simulink library "vmc"  (R2021b)
settings: Solver=VariableStepAuto  StartTime=0.0  StopTime=10.0  RelTol=1e-3
undefined symbols (not defined in the file or in its folder): AVMC_ACCDeltaTqIGain_X_kph, AVMC_ACCDeltaTqIGain_Y_mps2, AVMC_ACCDeltaTqPGain_X_kph, AVMC_ACCDeltaTqPGain_Y_kph, AVMC_ACCLongSteadyCtrl_X_kph, AVMC_AggressJerkPCT4AT_X_kph, AVMC_AggressJerkPCT_X_kph, AVMC_AggressLimitPCT4AT_X_kph, AVMC_AggressLimitPCT_X_kph, AVMC_CCLongSteadyCtrl_X_kph, AVMC_DISCDeltaTqIGain_X_kph, AVMC_DISCDeltaTqIGain_Y_mps2, AVMC_DISCDeltaTqPGain_X_kph, AVMC_DISCDeltaTqPGain_Y_kph, AVMC_DISCTrunAccJerk_X_s, AVMC_DISCTrunAccLimit_X_s, AVMC_ESCRegenOut_X_kph, AVMC_ESCRegenOut_Y_Deg, AVMC_ESCRegenOutEnSpd_X_Deg, AVMC_ISOAccLimit_X_mps, AVMC_ISODecLimit_X_mps, AVMC_ISOJerk_X_mps, AVMC_LatESCRegenOut_X_kph, AVMC_LatESCRegenOut_Y_Deg, AVMC_LongAccDeadZone_X_kph, AVMC_LongAccFiltTsforP2_X_Gps, AVMC_MCPresBaseTq_X_bar, AVMC_MSALongSteadyCtrl_X_kph, AVMC_MSAPedalOvrd2_X_kph, AVMC_MSAPedalOvrd_X_kph, AVMC_MSASpdBand_X_kph, AVMC_MSATqDownEndTq_X_kph, AVMC_MSATqDownTime_X_kph, AVMC_OPDDisSlideRate_X_Deg, AVMC_RDCDetectTime_X_kph, AVMC_RDCDetectTime_Y_pct, AVMC_RDCEnSlideRate_X_Deg, AVMC_RearWhlTqRatio_X_Nm, AVMC_RearWhlTqRatio_Y_gps, AVMC_RearWhlTqSlipGain_X_rat, AVMC_RearWhlTqSlipGain_Y_kph, AVMC_RearWhlTqSTRGGain_X_deg, AVMC_RearWhlTqSTRGGain_Y_kph, AVMC_RWSRrTSA2RWSPos_X_deg, AVMC_RWSSAS2FrtTSA_X_deg, AVMC_RWSVehSPD2RWSCoef_X_kph, AVMC_SoftJerkPCT_X_kph, AVMC_SoftLimitPCT_X_kph, AVMC_StESCYaw_X_kph, AVMC_StESCYaw_Y_Deg, AVMC_StESCYawCom_X_kph, AVMC_StESCYawCom_Y_Gps, AVMC_TMSpdBaseTq_X_rpm, AVMC_VehHoldBDecMap_X_kph, AVMC_VehHoldDecCtrlTime_X_kph, AVMC_VehHoldMCPPass_X_deg, C_TASK_10MS_S, C_TASK_5MS_S, DEG2RAD, ENUM_ACCAVAIL_AVAILABLE ... (+409)
libraries: hcu_lib x74, simulink x68, simulink_extras x3, $bdroot x2
(part 14 of 15)

== stateflow chart vmc/VMC/VMC/IMU/IMU sensing result /RollingAverage2 ==
  state RollingAverage
    (default) -> (junction 2) : {VVMC_RollAveCount_enum = ONE_INT}
    RollingAverage -> (junction 2)
    (junction 2) -> (junction 3) : {VVMC_RollAve_raw32 = ZERO_FLOAT}
    (junction 3) -> (junction 100) [order 1] : [VVMC_RollAveCount_enum < KVMC_RollAveLevel_enum]
    (junction 3) -> (junction 37) [order 2]
    (junction 100) -> (junction 5) : {% Memory
        |  VVMC_Memory_raw32[VVMC_RollAveCount_enum] = VINP_INPData_raw32;
        |
        |  % Memory Shift Counter
        |  VVMC_ShiftCount_enum = ONE_INT}
    (junction 5) -> (junction 7) [order 2]
    (junction 5) -> (junction 6) [order 1] : [VVMC_ShiftCount_enum <= VVMC_RollAveCount_enum]
    (junction 7) -> (junction 8) : {% Rolling Average
        |  VVMC_RollAve_raw32 = VVMC_RollAve_raw32 / VVMC_RollAveCount_enum;
        |
        |  % Rolling Average Counter
        |  VVMC_RollAveCount_enum++}
    (junction 35) -> (junction 5) : {VVMC_ShiftCount_enum++}
    (junction 6) -> (junction 36) : {% Rolling Average Sum
        |  VVMC_RollAve_raw32 = VVMC_RollAve_raw32 + VVMC_Memory_raw32[VVMC_ShiftCount_enum];
        |  }
    (junction 36) -> (junction 35)
    (junction 37) -> (junction 76) [order 1] : [VVMC_RollAveCount_enum == KVMC_RollAveLevel_enum]
    (junction 76) -> (junction 47)
    (junction 37) -> (junction 60) [order 2]
    (junction 78) -> (junction 76)
    (junction 47) -> (junction 30) : {% Memory
        |  VVMC_Memory_raw32[VVMC_RollAveCount_enum] = VINP_INPData_raw32;
        |
        |  % Memory Shift Counter
        |  VVMC_ShiftCount_enum = ONE_INT;
        | }
    (junction 60) -> (junction 62) [order 1] : [VVMC_RollAveCount_enum > KVMC_RollAveLevel_enum]
    (junction 60) -> (junction 39) [order 2]
    (junction 62) -> (junction 66) : {VVMC_MemoryShiftCount_enum = ONE_INT}
    (junction 30) -> (junction 48) [order 2]
    (junction 30) -> (junction 22) [order 1] : [VVMC_ShiftCount_enum <= VVMC_RollAveCount_enum]
    (junction 48) -> (junction 45) : {% Rolling Average
        |  VVMC_RollAve_raw32 = VVMC_RollAve_raw32 / VVMC_RollAveCount_enum;
        |
        |  % Memory Shift Counter
        |  VVMC_ShiftCount_enum = ONE_INT}
    (junction 14) -> (junction 30) : {VVMC_ShiftCount_enum++}
    (junction 22) -> (junction 25) : {% Rolling Average Sum
        |  VVMC_RollAve_raw32 = VVMC_RollAve_raw32 + VVMC_Memory_raw32[VVMC_ShiftCount_enum]}
    (junction 66) -> (junction 82) [order 2]
    (junction 66) -> (junction 69) [order 1] : [VVMC_MemoryShiftCount_enum < VVMC_RollAveCount_enum]
    (junction 82) -> (junction 80) : {VVMC_RollAveCount_enum = KVMC_RollAveLevel_enum}
    (junction 73) -> (junction 66) : {VVMC_MemoryShiftCount_enum++}
    (junction 69) -> (junction 71) : {VVMC_Memory_raw32[VVMC_MemoryShiftCount_enum] =...
        |  VVMC_Memory_raw32[VVMC_RollAveCount_enum - KVMC_RollAveLevel_enum + VVMC_MemoryShiftCount_enum]}
    (junction 25) -> (junction 14)
    (junction 71) -> (junction 73)
    (junction 80) -> (junction 78)
    (junction 45) -> (junction 39) [order 2]
    (junction 45) -> (junction 15) [order 1] : [VVMC_ShiftCount_enum < VVMC_RollAveCount_enum]
    (junction 41) -> (junction 45) : { VVMC_ShiftCount_enum++}
    (junction 15) -> (junction 38) : {% Gy Memory Shift
        |  VVMC_Memory_raw32[VVMC_ShiftCount_enum] = VVMC_Memory_raw32[VVMC_ShiftCount_enum + ONE_INT]}
    (junction 38) -> (junction 41)
  data: KVMC_RollAveLevel_enum input uint8; VVMC_ShiftCount_enum local uint8; VVMC_RollAveCount_enum local uint8; VVMC_Memory_raw32 local single size=100; ZERO_FLOAT input single; ONE_INT input uint8; VVMC_RollAve_raw32 output single; VINP_INPData_raw32 input single; VVMC_MemoryShiftCount_enum local uint8

== stateflow chart vmc/VMC/VMC/IMU/IMU sensing result /RollingAverage3 ==
  state RollingAverage
    (default) -> (junction 2) : {VVMC_RollAveCount_enum = ONE_INT}
    RollingAverage -> (junction 2)
    (junction 2) -> (junction 3) : {VVMC_RollAve_raw32 = ZERO_FLOAT}
    (junction 3) -> (junction 100) [order 1] : [VVMC_RollAveCount_enum < KVMC_RollAveLevel_enum]
    (junction 3) -> (junction 37) [order 2]
    (junction 100) -> (junction 5) : {% Memory
        |  VVMC_Memory_raw32[VVMC_RollAveCount_enum] = VINP_INPData_raw32;
        |
        |  % Memory Shift Counter
        |  VVMC_ShiftCount_enum = ONE_INT}
    (junction 5) -> (junction 7) [order 2]
    (junction 5) -> (junction 6) [order 1] : [VVMC_ShiftCount_enum <= VVMC_RollAveCount_enum]
    (junction 7) -> (junction 8) : {% Rolling Average
        |  VVMC_RollAve_raw32 = VVMC_RollAve_raw32 / VVMC_RollAveCount_enum;
        |
        |  % Rolling Average Counter
        |  VVMC_RollAveCount_enum++}
    (junction 35) -> (junction 5) : {VVMC_ShiftCount_enum++}
    (junction 6) -> (junction 36) : {% Rolling Average Sum
        |  VVMC_RollAve_raw32 = VVMC_RollAve_raw32 + VVMC_Memory_raw32[VVMC_ShiftCount_enum];
        |  }
    (junction 36) -> (junction 35)
    (junction 37) -> (junction 76) [order 1] : [VVMC_RollAveCount_enum == KVMC_RollAveLevel_enum]
    (junction 76) -> (junction 47)
    (junction 37) -> (junction 60) [order 2]
    (junction 78) -> (junction 76)
    (junction 47) -> (junction 30) : {% Memory
        |  VVMC_Memory_raw32[VVMC_RollAveCount_enum] = VINP_INPData_raw32;
        |
        |  % Memory Shift Counter
        |  VVMC_ShiftCount_enum = ONE_INT;
        | }
    (junction 60) -> (junction 62) [order 1] : [VVMC_RollAveCount_enum > KVMC_RollAveLevel_enum]
    (junction 60) -> (junction 39) [order 2]
    (junction 62) -> (junction 66) : {VVMC_MemoryShiftCount_enum = ONE_INT}
    (junction 30) -> (junction 48) [order 2]
    (junction 30) -> (junction 22) [order 1] : [VVMC_ShiftCount_enum <= VVMC_RollAveCount_enum]
    (junction 48) -> (junction 45) : {% Rolling Average
        |  VVMC_RollAve_raw32 = VVMC_RollAve_raw32 / VVMC_RollAveCount_enum;
        |
        |  % Memory Shift Counter
        |  VVMC_ShiftCount_enum = ONE_INT}
    (junction 14) -> (junction 30) : {VVMC_ShiftCount_enum++}
    (junction 22) -> (junction 25) : {% Rolling Average Sum
        |  VVMC_RollAve_raw32 = VVMC_RollAve_raw32 + VVMC_Memory_raw32[VVMC_ShiftCount_enum]}
    (junction 66) -> (junction 82) [order 2]
    (junction 66) -> (junction 69) [order 1] : [VVMC_MemoryShiftCount_enum < VVMC_RollAveCount_enum]
    (junction 82) -> (junction 80) : {VVMC_RollAveCount_enum = KVMC_RollAveLevel_enum}
    (junction 73) -> (junction 66) : {VVMC_MemoryShiftCount_enum++}
    (junction 69) -> (junction 71) : {VVMC_Memory_raw32[VVMC_MemoryShiftCount_enum] =...
        |  VVMC_Memory_raw32[VVMC_RollAveCount_enum - KVMC_RollAveLevel_enum + VVMC_MemoryShiftCount_enum]}
    (junction 25) -> (junction 14)
    (junction 71) -> (junction 73)
    (junction 80) -> (junction 78)
    (junction 45) -> (junction 39) [order 2]
    (junction 45) -> (junction 15) [order 1] : [VVMC_ShiftCount_enum < VVMC_RollAveCount_enum]
    (junction 41) -> (junction 45) : { VVMC_ShiftCount_enum++}
    (junction 15) -> (junction 38) : {% Gy Memory Shift
        |  VVMC_Memory_raw32[VVMC_ShiftCount_enum] = VVMC_Memory_raw32[VVMC_ShiftCount_enum + ONE_INT]}
    (junction 38) -> (junction 41)
  data: KVMC_RollAveLevel_enum input uint8; VVMC_ShiftCount_enum local uint8; VVMC_RollAveCount_enum local uint8; VVMC_Memory_raw32 local single size=100; ZERO_FLOAT input single; ONE_INT input uint8; VVMC_RollAve_raw32 output single; VINP_INPData_raw32 input single; VVMC_MemoryShiftCount_enum local uint8

== stateflow chart vmc/VMC/VMC/SafetyControl/VehSpdRollingAverage/RollingAverage ==
  state LatAccelRollingAverage
    (default) -> (junction 2) : {VVMC_RollAveCount_enum = ONE_INT}
    LatAccelRollingAverage -> (junction 2)
    (junction 2) -> (junction 3) : {VVMC_VehSpdRollAve_kph = ZERO_FLOAT}
    (junction 3) -> (junction 100) [order 1] : [VVMC_RollAveCount_enum < KVMC_VehSpdRollAveLevel_enum]
    (junction 3) -> (junction 37) [order 2]
    (junction 100) -> (junction 5) : {% Memory
        |  VVMC_Memory_raw32[VVMC_RollAveCount_enum] = VINP_VehSpeed_kph;
        |
        |  % Memory Shift Counter
        |  VVMC_ShiftCount_enum = ONE_INT}
    (junction 5) -> (junction 7) [order 2]
    (junction 5) -> (junction 6) [order 1] : [VVMC_ShiftCount_enum <= VVMC_RollAveCount_enum]
    (junction 7) -> (junction 8) : {% Rolling Average
        |  VVMC_VehSpdRollAve_kph = VVMC_VehSpdRollAve_kph / VVMC_RollAveCount_enum;
        |
        |  % Rolling Average Counter
        |  VVMC_RollAveCount_enum++}
    (junction 35) -> (junction 5) : {VVMC_ShiftCount_enum++}
    (junction 6) -> (junction 36) : {% Rolling Average Sum
        |  VVMC_VehSpdRollAve_kph = VVMC_VehSpdRollAve_kph + VVMC_Memory_raw32[VVMC_ShiftCount_enum];
        |  }
    (junction 36) -> (junction 35)
    (junction 37) -> (junction 76) [order 1] : [VVMC_RollAveCount_enum == KVMC_VehSpdRollAveLevel_enum]
    (junction 76) -> (junction 47)
    (junction 37) -> (junction 60) [order 2]
    (junction 78) -> (junction 76)
    (junction 47) -> (junction 30) : {% Memory
        |  VVMC_Memory_raw32[VVMC_RollAveCount_enum] = VINP_VehSpeed_kph;
        |
        |  % Memory Shift Counter
        |  VVMC_ShiftCount_enum = ONE_INT;
        | }
    (junction 60) -> (junction 62) [order 1] : [VVMC_RollAveCount_enum > KVMC_VehSpdRollAveLevel_enum]
    (junction 60) -> (junction 39) [order 2]
    (junction 62) -> (junction 66) : {VVMC_MemoryShiftCount_enum = ONE_INT}
    (junction 30) -> (junction 48) [order 2]
    (junction 30) -> (junction 22) [order 1] : [VVMC_ShiftCount_enum <= VVMC_RollAveCount_enum]
    (junction 48) -> (junction 45) : {% Rolling Average
        |  VVMC_VehSpdRollAve_kph = VVMC_VehSpdRollAve_kph / VVMC_RollAveCount_enum;
        |
        |  % Memory Shift Counter
        |  VVMC_ShiftCount_enum = ONE_INT}
    (junction 14) -> (junction 30) : {VVMC_ShiftCount_enum++}
    (junction 22) -> (junction 25) : {% Rolling Average Sum
        |  VVMC_VehSpdRollAve_kph = VVMC_VehSpdRollAve_kph + VVMC_Memory_raw32[VVMC_ShiftCount_enum]}
    (junction 66) -> (junction 82) [order 2]
    (junction 66) -> (junction 69) [order 1] : [VVMC_MemoryShiftCount_enum < VVMC_RollAveCount_enum]
    (junction 82) -> (junction 80) : {VVMC_RollAveCount_enum = KVMC_VehSpdRollAveLevel_enum}
    (junction 73) -> (junction 66) : {VVMC_MemoryShiftCount_enum++}
    (junction 69) -> (junction 71) : {VVMC_Memory_raw32[VVMC_MemoryShiftCount_enum] =...
        |  VVMC_Memory_raw32[VVMC_RollAveCount_enum - KVMC_VehSpdRollAveLevel_enum + VVMC_MemoryShiftCount_enum]}
    (junction 25) -> (junction 14)
    (junction 71) -> (junction 73)
    (junction 80) -> (junction 78)
    (junction 45) -> (junction 39) [order 2]
    (junction 45) -> (junction 15) [order 1] : [VVMC_ShiftCount_enum < VVMC_RollAveCount_enum]
    (junction 41) -> (junction 45) : { VVMC_ShiftCount_enum++}
    (junction 15) -> (junction 38) : {% Gy Memory Shift
        |  VVMC_Memory_raw32[VVMC_ShiftCount_enum] = VVMC_Memory_raw32[VVMC_ShiftCount_enum + ONE_INT]}
    (junction 38) -> (junction 41)
  data: KVMC_VehSpdRollAveLevel_enum input uint8; VVMC_ShiftCount_enum local uint8; VVMC_RollAveCount_enum local uint8; VVMC_Memory_raw32 local single size=100; ZERO_FLOAT input single; ONE_INT input uint8; VVMC_VehSpdRollAve_kph output single; VINP_VehSpeed_kph input single; VVMC_MemoryShiftCount_enum local uint8

== stateflow chart vmc/VMC/VMC/SpeedCalculation/RollingAverage ==
  state LatAccelRollingAverage
    (default) -> (junction 2) : {VVMC_RollAveCount_enum = ONE_INT}
    LatAccelRollingAverage -> (junction 2)
    (junction 2) -> (junction 3) : {VVMC_MeterSpdRollAve_kph = ZERO_FLOAT}
    (junction 3) -> (junction 100) [order 1] : [VVMC_RollAveCount_enum < KVMC_MeterSpdRollAveLevel_enum]
    (junction 3) -> (junction 37) [order 2]
    (junction 100) -> (junction 5) : {% Memory
        |  VVMC_Memory_raw32[VVMC_RollAveCount_enum] = VINP_MeterIndVehSpeed_kph;
        |
        |  % Memory Shift Counter
        |  VVMC_ShiftCount_enum = ONE_INT}
    (junction 5) -> (junction 7) [order 2]
    (junction 5) -> (junction 6) [order 1] : [VVMC_ShiftCount_enum <= VVMC_RollAveCount_enum]
    (junction 7) -> (junction 8) : {% Rolling Average
        |  VVMC_MeterSpdRollAve_kph = VVMC_MeterSpdRollAve_kph / VVMC_RollAveCount_enum;
        |
        |  % Rolling Average Counter
        |  VVMC_RollAveCount_enum++}
    (junction 35) -> (junction 5) : {VVMC_ShiftCount_enum++}
    (junction 6) -> (junction 36) : {% Rolling Average Sum
        |  VVMC_MeterSpdRollAve_kph = VVMC_MeterSpdRollAve_kph + VVMC_Memory_raw32[VVMC_ShiftCount_enum];
        |  }
    (junction 36) -> (junction 35)
    (junction 37) -> (junction 76) [order 1] : [VVMC_RollAveCount_enum == KVMC_MeterSpdRollAveLevel_enum]
    (junction 76) -> (junction 47)
    (junction 37) -> (junction 60) [order 2]
    (junction 78) -> (junction 76)
    (junction 47) -> (junction 30) : {% Memory
        |  VVMC_Memory_raw32[VVMC_RollAveCount_enum] = VINP_MeterIndVehSpeed_kph;
        |
        |  % Memory Shift Counter
        |  VVMC_ShiftCount_enum = ONE_INT;
        | }
    (junction 60) -> (junction 62) [order 1] : [VVMC_RollAveCount_enum > KVMC_MeterSpdRollAveLevel_enum]
    (junction 60) -> (junction 39) [order 2]
    (junction 62) -> (junction 66) : {VVMC_MemoryShiftCount_enum = ONE_INT}
    (junction 30) -> (junction 48) [order 2]
    (junction 30) -> (junction 22) [order 1] : [VVMC_ShiftCount_enum <= VVMC_RollAveCount_enum]
    (junction 48) -> (junction 45) : {% Rolling Average
        |  VVMC_MeterSpdRollAve_kph = VVMC_MeterSpdRollAve_kph / VVMC_RollAveCount_enum;
        |
        |  % Memory Shift Counter
        |  VVMC_ShiftCount_enum = ONE_INT}
    (junction 14) -> (junction 30) : {VVMC_ShiftCount_enum++}
    (junction 22) -> (junction 25) : {% Rolling Average Sum
        |  VVMC_MeterSpdRollAve_kph = VVMC_MeterSpdRollAve_kph + VVMC_Memory_raw32[VVMC_ShiftCount_enum]}
    (junction 66) -> (junction 82) [order 2]
    (junction 66) -> (junction 69) [order 1] : [VVMC_MemoryShiftCount_enum < VVMC_RollAveCount_enum]
    (junction 82) -> (junction 80) : {VVMC_RollAveCount_enum = KVMC_MeterSpdRollAveLevel_enum}
    (junction 73) -> (junction 66) : {VVMC_MemoryShiftCount_enum++}
    (junction 69) -> (junction 71) : {VVMC_Memory_raw32[VVMC_MemoryShiftCount_enum] =...
        |  VVMC_Memory_raw32[VVMC_RollAveCount_enum - KVMC_MeterSpdRollAveLevel_enum + VVMC_MemoryShiftCount_enum]}
    (junction 25) -> (junction 14)
    (junction 71) -> (junction 73)
    (junction 80) -> (junction 78)
    (junction 45) -> (junction 39) [order 2]
    (junction 45) -> (junction 15) [order 1] : [VVMC_ShiftCount_enum < VVMC_RollAveCount_enum]
    (junction 41) -> (junction 45) : { VVMC_ShiftCount_enum++}
    (junction 15) -> (junction 38) : {% Gy Memory Shift
        |  VVMC_Memory_raw32[VVMC_ShiftCount_enum] = VVMC_Memory_raw32[VVMC_ShiftCount_enum + ONE_INT]}
    (junction 38) -> (junction 41)
  data: KVMC_MeterSpdRollAveLevel_enum input uint8; VVMC_ShiftCount_enum local uint8; VVMC_RollAveCount_enum local uint8; VVMC_Memory_raw32 local single size=300; ZERO_FLOAT input single; ONE_INT input uint8; VVMC_MeterSpdRollAve_kph output single; VINP_MeterIndVehSpeed_kph input single; VVMC_MemoryShiftCount_enum local uint8

== stateflow chart vmc/VMC/VMC/SafetyControl/WheelSpeedRollingAverage/RollingAverage ==
  state LatAccelRollingAverage
    (default) -> (junction 2) : {VVMC_RollAveCount_enum = ONE_INT}
    LatAccelRollingAverage -> (junction 2)
    (junction 2) -> (junction 3) : {VVMC_LFWhlSpeedRollAve_kph = ZERO_FLOAT}
    (junction 3) -> (junction 100) [order 1] : [VVMC_RollAveCount_enum < KVMC_WhlSpdRollAveLevel_enum]
    (junction 3) -> (junction 37) [order 2]
    (junction 100) -> (junction 5) : {% Memory
        |  VVMC_Memory_raw32[VVMC_RollAveCount_enum] = VINP_LFRawWhlSpeed_kph;
        |
        |  % Memory Shift Counter
        |  VVMC_ShiftCount_enum = ONE_INT}
    (junction 5) -> (junction 7) [order 2]
    (junction 5) -> (junction 6) [order 1] : [VVMC_ShiftCount_enum <= VVMC_RollAveCount_enum]
    (junction 7) -> (junction 8) : {% Rolling Average
        |  VVMC_LFWhlSpeedRollAve_kph = VVMC_LFWhlSpeedRollAve_kph / VVMC_RollAveCount_enum;
        |
        |  % Rolling Average Counter
        |  VVMC_RollAveCount_enum++}
    (junction 35) -> (junction 5) : {VVMC_ShiftCount_enum++}
    (junction 6) -> (junction 36) : {% Rolling Average Sum
        |  VVMC_LFWhlSpeedRollAve_kph = VVMC_LFWhlSpeedRollAve_kph + VVMC_Memory_raw32[VVMC_ShiftCount_enum];
        |  }
    (junction 36) -> (junction 35)
    (junction 37) -> (junction 76) [order 1] : [VVMC_RollAveCount_enum == KVMC_WhlSpdRollAveLevel_enum]
    (junction 76) -> (junction 47)
    (junction 37) -> (junction 60) [order 2]
    (junction 78) -> (junction 76)
    (junction 47) -> (junction 30) : {% Memory
        |  VVMC_Memory_raw32[VVMC_RollAveCount_enum] = VINP_LFRawWhlSpeed_kph;
        |
        |  % Memory Shift Counter
        |  VVMC_ShiftCount_enum = ONE_INT;
        | }
    (junction 60) -> (junction 62) [order 1] : [VVMC_RollAveCount_enum > KVMC_WhlSpdRollAveLevel_enum]
    (junction 60) -> (junction 39) [order 2]
    (junction 62) -> (junction 66) : {VVMC_MemoryShiftCount_enum = ONE_INT}
    (junction 30) -> (junction 48) [order 2]
    (junction 30) -> (junction 22) [order 1] : [VVMC_ShiftCount_enum <= VVMC_RollAveCount_enum]
    (junction 48) -> (junction 45) : {% Rolling Average
        |  VVMC_LFWhlSpeedRollAve_kph = VVMC_LFWhlSpeedRollAve_kph / VVMC_RollAveCount_enum;
        |
        |  % Memory Shift Counter
        |  VVMC_ShiftCount_enum = ONE_INT}
    (junction 14) -> (junction 30) : {VVMC_ShiftCount_enum++}
    (junction 22) -> (junction 25) : {% Rolling Average Sum
        |  VVMC_LFWhlSpeedRollAve_kph = VVMC_LFWhlSpeedRollAve_kph + VVMC_Memory_raw32[VVMC_ShiftCount_enum]}
    (junction 66) -> (junction 82) [order 2]
    (junction 66) -> (junction 69) [order 1] : [VVMC_MemoryShiftCount_enum < VVMC_RollAveCount_enum]
    (junction 82) -> (junction 80) : {VVMC_RollAveCount_enum = KVMC_WhlSpdRollAveLevel_enum}
    (junction 73) -> (junction 66) : {VVMC_MemoryShiftCount_enum++}
    (junction 69) -> (junction 71) : {VVMC_Memory_raw32[VVMC_MemoryShiftCount_enum] =...
        |  VVMC_Memory_raw32[VVMC_RollAveCount_enum - KVMC_WhlSpdRollAveLevel_enum + VVMC_MemoryShiftCount_enum]}
    (junction 25) -> (junction 14)
    (junction 71) -> (junction 73)
    (junction 80) -> (junction 78)
    (junction 45) -> (junction 39) [order 2]
    (junction 45) -> (junction 15) [order 1] : [VVMC_ShiftCount_enum < VVMC_RollAveCount_enum]
    (junction 41) -> (junction 45) : { VVMC_ShiftCount_enum++}
    (junction 15) -> (junction 38) : {% Gy Memory Shift
        |  VVMC_Memory_raw32[VVMC_ShiftCount_enum] = VVMC_Memory_raw32[VVMC_ShiftCount_enum + ONE_INT]}
    (junction 38) -> (junction 41)
  data: KVMC_WhlSpdRollAveLevel_enum input uint8; VVMC_ShiftCount_enum local uint8; VVMC_RollAveCount_enum local uint8; VVMC_Memory_raw32 local single size=100; ZERO_FLOAT input single; ONE_INT input uint8; VVMC_LFWhlSpeedRollAve_kph output single; VINP_LFRawWhlSpeed_kph input single; VVMC_MemoryShiftCount_enum local uint8

== stateflow chart vmc/VMC/VMC/SafetyControl/WheelSpeedRollingAverage/RollingAverage1 ==
  state LatAccelRollingAverage
    (default) -> (junction 2) : {VVMC_RollAveCount_enum = ONE_INT}
    LatAccelRollingAverage -> (junction 2)
    (junction 2) -> (junction 3) : {VVMC_RFWhlSpeedRollAve_kph = ZERO_FLOAT}
    (junction 3) -> (junction 100) [order 1] : [VVMC_RollAveCount_enum < KVMC_WhlSpdRollAveLevel_enum]
    (junction 3) -> (junction 37) [order 2]
    (junction 100) -> (junction 5) : {% Memory
        |  VVMC_Memory_raw32[VVMC_RollAveCount_enum] = VINP_RFRawWhlSpeed_kph;
        |
        |  % Memory Shift Counter
        |  VVMC_ShiftCount_enum = ONE_INT}
    (junction 5) -> (junction 7) [order 2]
    (junction 5) -> (junction 6) [order 1] : [VVMC_ShiftCount_enum <= VVMC_RollAveCount_enum]
    (junction 7) -> (junction 8) : {% Rolling Average
        |  VVMC_RFWhlSpeedRollAve_kph = VVMC_RFWhlSpeedRollAve_kph / VVMC_RollAveCount_enum;
        |
        |  % Rolling Average Counter
        |  VVMC_RollAveCount_enum++}
    (junction 35) -> (junction 5) : {VVMC_ShiftCount_enum++}
    (junction 6) -> (junction 36) : {% Rolling Average Sum
        |  VVMC_RFWhlSpeedRollAve_kph = VVMC_RFWhlSpeedRollAve_kph + VVMC_Memory_raw32[VVMC_ShiftCount_enum];
        |  }
    (junction 36) -> (junction 35)
    (junction 37) -> (junction 76) [order 1] : [VVMC_RollAveCount_enum == KVMC_WhlSpdRollAveLevel_enum]
    (junction 76) -> (junction 47)
    (junction 37) -> (junction 60) [order 2]
    (junction 78) -> (junction 76)
    (junction 47) -> (junction 30) : {% Memory
        |  VVMC_Memory_raw32[VVMC_RollAveCount_enum] = VINP_RFRawWhlSpeed_kph;
        |
        |  % Memory Shift Counter
        |  VVMC_ShiftCount_enum = ONE_INT;
        | }
    (junction 60) -> (junction 62) [order 1] : [VVMC_RollAveCount_enum > KVMC_WhlSpdRollAveLevel_enum]
    (junction 60) -> (junction 39) [order 2]
    (junction 62) -> (junction 66) : {VVMC_MemoryShiftCount_enum = ONE_INT}
    (junction 30) -> (junction 48) [order 2]
    (junction 30) -> (junction 22) [order 1] : [VVMC_ShiftCount_enum <= VVMC_RollAveCount_enum]
    (junction 48) -> (junction 45) : {% Rolling Average
        |  VVMC_RFWhlSpeedRollAve_kph = VVMC_RFWhlSpeedRollAve_kph / VVMC_RollAveCount_enum;
        |
        |  % Memory Shift Counter
        |  VVMC_ShiftCount_enum = ONE_INT}
    (junction 14) -> (junction 30) : {VVMC_ShiftCount_enum++}
    (junction 22) -> (junction 25) : {% Rolling Average Sum
        |  VVMC_RFWhlSpeedRollAve_kph = VVMC_RFWhlSpeedRollAve_kph + VVMC_Memory_raw32[VVMC_ShiftCount_enum]}
    (junction 66) -> (junction 82) [order 2]
    (junction 66) -> (junction 69) [order 1] : [VVMC_MemoryShiftCount_enum < VVMC_RollAveCount_enum]
    (junction 82) -> (junction 80) : {VVMC_RollAveCount_enum = KVMC_WhlSpdRollAveLevel_enum}
    (junction 73) -> (junction 66) : {VVMC_MemoryShiftCount_enum++}
    (junction 69) -> (junction 71) : {VVMC_Memory_raw32[VVMC_MemoryShiftCount_enum] =...
        |  VVMC_Memory_raw32[VVMC_RollAveCount_enum - KVMC_WhlSpdRollAveLevel_enum + VVMC_MemoryShiftCount_enum]}
    (junction 25) -> (junction 14)
    (junction 71) -> (junction 73)
    (junction 80) -> (junction 78)
    (junction 45) -> (junction 39) [order 2]
    (junction 45) -> (junction 15) [order 1] : [VVMC_ShiftCount_enum < VVMC_RollAveCount_enum]
    (junction 41) -> (junction 45) : { VVMC_ShiftCount_enum++}
    (junction 15) -> (junction 38) : {% Gy Memory Shift
        |  VVMC_Memory_raw32[VVMC_ShiftCount_enum] = VVMC_Memory_raw32[VVMC_ShiftCount_enum + ONE_INT]}
    (junction 38) -> (junction 41)
  data: KVMC_WhlSpdRollAveLevel_enum input uint8; VVMC_ShiftCount_enum local uint8; VVMC_RollAveCount_enum local uint8; VVMC_Memory_raw32 local single size=100; ZERO_FLOAT input single; ONE_INT input uint8; VVMC_RFWhlSpeedRollAve_kph output single; VINP_RFRawWhlSpeed_kph input single; VVMC_MemoryShiftCount_enum local uint8

== stateflow chart vmc/VMC/VMC/SafetyControl/WheelSpeedRollingAverage/RollingAverage2 ==
  state LatAccelRollingAverage
    (default) -> (junction 2) : {VVMC_RollAveCount_enum = ONE_INT}
    LatAccelRollingAverage -> (junction 2)
    (junction 2) -> (junction 3) : {VVMC_LRWhlSpeedRollAve_kph = ZERO_FLOAT}
    (junction 3) -> (junction 100) [order 1] : [VVMC_RollAveCount_enum < KVMC_WhlSpdRollAveLevel_enum]
    (junction 3) -> (junction 37) [order 2]
    (junction 100) -> (junction 5) : {% Memory
        |  VVMC_Memory_raw32[VVMC_RollAveCount_enum] = VINP_LRRawWhlSpeed_kph;
        |
        |  % Memory Shift Counter
        |  VVMC_ShiftCount_enum = ONE_INT}
    (junction 5) -> (junction 7) [order 2]
    (junction 5) -> (junction 6) [order 1] : [VVMC_ShiftCount_enum <= VVMC_RollAveCount_enum]
    (junction 7) -> (junction 8) : {% Rolling Average
        |  VVMC_LRWhlSpeedRollAve_kph = VVMC_LRWhlSpeedRollAve_kph / VVMC_RollAveCount_enum;
        |
        |  % Rolling Average Counter
        |  VVMC_RollAveCount_enum++}
    (junction 35) -> (junction 5) : {VVMC_ShiftCount_enum++}
    (junction 6) -> (junction 36) : {% Rolling Average Sum
        |  VVMC_LRWhlSpeedRollAve_kph = VVMC_LRWhlSpeedRollAve_kph + VVMC_Memory_raw32[VVMC_ShiftCount_enum];
        |  }
    (junction 36) -> (junction 35)
    (junction 37) -> (junction 76) [order 1] : [VVMC_RollAveCount_enum == KVMC_WhlSpdRollAveLevel_enum]
    (junction 76) -> (junction 47)
    (junction 37) -> (junction 60) [order 2]
    (junction 78) -> (junction 76)
    (junction 47) -> (junction 30) : {% Memory
        |  VVMC_Memory_raw32[VVMC_RollAveCount_enum] = VINP_LRRawWhlSpeed_kph;
        |
        |  % Memory Shift Counter
        |  VVMC_ShiftCount_enum = ONE_INT;
        | }
    (junction 60) -> (junction 62) [order 1] : [VVMC_RollAveCount_enum > KVMC_WhlSpdRollAveLevel_enum]
    (junction 60) -> (junction 39) [order 2]
    (junction 62) -> (junction 66) : {VVMC_MemoryShiftCount_enum = ONE_INT}
    (junction 30) -> (junction 48) [order 2]
    (junction 30) -> (junction 22) [order 1] : [VVMC_ShiftCount_enum <= VVMC_RollAveCount_enum]
    (junction 48) -> (junction 45) : {% Rolling Average
        |  VVMC_LRWhlSpeedRollAve_kph = VVMC_LRWhlSpeedRollAve_kph / VVMC_RollAveCount_enum;
        |
        |  % Memory Shift Counter
        |  VVMC_ShiftCount_enum = ONE_INT}
    (junction 14) -> (junction 30) : {VVMC_ShiftCount_enum++}
    (junction 22) -> (junction 25) : {% Rolling Average Sum
        |  VVMC_LRWhlSpeedRollAve_kph = VVMC_LRWhlSpeedRollAve_kph + VVMC_Memory_raw32[VVMC_ShiftCount_enum]}
    (junction 66) -> (junction 82) [order 2]
    (junction 66) -> (junction 69) [order 1] : [VVMC_MemoryShiftCount_enum < VVMC_RollAveCount_enum]
    (junction 82) -> (junction 80) : {VVMC_RollAveCount_enum = KVMC_WhlSpdRollAveLevel_enum}
    (junction 73) -> (junction 66) : {VVMC_MemoryShiftCount_enum++}
    (junction 69) -> (junction 71) : {VVMC_Memory_raw32[VVMC_MemoryShiftCount_enum] =...
        |  VVMC_Memory_raw32[VVMC_RollAveCount_enum - KVMC_WhlSpdRollAveLevel_enum + VVMC_MemoryShiftCount_enum]}
    (junction 25) -> (junction 14)
    (junction 71) -> (junction 73)
    (junction 80) -> (junction 78)
    (junction 45) -> (junction 39) [order 2]
    (junction 45) -> (junction 15) [order 1] : [VVMC_ShiftCount_enum < VVMC_RollAveCount_enum]
    (junction 41) -> (junction 45) : { VVMC_ShiftCount_enum++}
    (junction 15) -> (junction 38) : {% Gy Memory Shift
        |  VVMC_Memory_raw32[VVMC_ShiftCount_enum] = VVMC_Memory_raw32[VVMC_ShiftCount_enum + ONE_INT]}
    (junction 38) -> (junction 41)
  data: KVMC_WhlSpdRollAveLevel_enum input uint8; VVMC_ShiftCount_enum local uint8; VVMC_RollAveCount_enum local uint8; VVMC_Memory_raw32 local single size=100; ZERO_FLOAT input single; ONE_INT input uint8; VVMC_LRWhlSpeedRollAve_kph output single; VINP_LRRawWhlSpeed_kph input single; VVMC_MemoryShiftCount_enum local uint8

== stateflow chart vmc/VMC/VMC/SafetyControl/WheelSpeedRollingAverage/RollingAverage3 ==
  state LatAccelRollingAverage
    (default) -> (junction 2) : {VVMC_RollAveCount_enum = ONE_INT}
    LatAccelRollingAverage -> (junction 2)
    (junction 2) -> (junction 3) : {VVMC_RRWhlSpeedRollAve_kph = ZERO_FLOAT}
    (junction 3) -> (junction 100) [order 1] : [VVMC_RollAveCount_enum < KVMC_WhlSpdRollAveLevel_enum]
    (junction 3) -> (junction 37) [order 2]
    (junction 100) -> (junction 5) : {% Memory
        |  VVMC_Memory_raw32[VVMC_RollAveCount_enum] = VINP_RRRawWhlSpeed_kph;
        |
        |  % Memory Shift Counter
        |  VVMC_ShiftCount_enum = ONE_INT}
    (junction 5) -> (junction 7) [order 2]
    (junction 5) -> (junction 6) [order 1] : [VVMC_ShiftCount_enum <= VVMC_RollAveCount_enum]
    (junction 7) -> (junction 8) : {% Rolling Average
        |  VVMC_RRWhlSpeedRollAve_kph = VVMC_RRWhlSpeedRollAve_kph / VVMC_RollAveCount_enum;
        |
        |  % Rolling Average Counter
        |  VVMC_RollAveCount_enum++}
    (junction 35) -> (junction 5) : {VVMC_ShiftCount_enum++}
    (junction 6) -> (junction 36) : {% Rolling Average Sum
        |  VVMC_RRWhlSpeedRollAve_kph = VVMC_RRWhlSpeedRollAve_kph + VVMC_Memory_raw32[VVMC_ShiftCount_enum];
        |  }
    (junction 36) -> (junction 35)
    (junction 37) -> (junction 76) [order 1] : [VVMC_RollAveCount_enum == KVMC_WhlSpdRollAveLevel_enum]
    (junction 76) -> (junction 47)
    (junction 37) -> (junction 60) [order 2]
    (junction 78) -> (junction 76)
    (junction 47) -> (junction 30) : {% Memory
        |  VVMC_Memory_raw32[VVMC_RollAveCount_enum] = VINP_RRRawWhlSpeed_kph;
        |
        |  % Memory Shift Counter
        |  VVMC_ShiftCount_enum = ONE_INT;
        | }
    (junction 60) -> (junction 62) [order 1] : [VVMC_RollAveCount_enum > KVMC_WhlSpdRollAveLevel_enum]
    (junction 60) -> (junction 39) [order 2]
    (junction 62) -> (junction 66) : {VVMC_MemoryShiftCount_enum = ONE_INT}
    (junction 30) -> (junction 48) [order 2]
    (junction 30) -> (junction 22) [order 1] : [VVMC_ShiftCount_enum <= VVMC_RollAveCount_enum]
    (junction 48) -> (junction 45) : {% Rolling Average
        |  VVMC_RRWhlSpeedRollAve_kph = VVMC_RRWhlSpeedRollAve_kph / VVMC_RollAveCount_enum;
        |
        |  % Memory Shift Counter
        |  VVMC_ShiftCount_enum = ONE_INT}
    (junction 14) -> (junction 30) : {VVMC_ShiftCount_enum++}
    (junction 22) -> (junction 25) : {% Rolling Average Sum
        |  VVMC_RRWhlSpeedRollAve_kph = VVMC_RRWhlSpeedRollAve_kph + VVMC_Memory_raw32[VVMC_ShiftCount_enum]}
    (junction 66) -> (junction 82) [order 2]
    (junction 66) -> (junction 69) [order 1] : [VVMC_MemoryShiftCount_enum < VVMC_RollAveCount_enum]
    (junction 82) -> (junction 80) : {VVMC_RollAveCount_enum = KVMC_WhlSpdRollAveLevel_enum}
    (junction 73) -> (junction 66) : {VVMC_MemoryShiftCount_enum++}
    (junction 69) -> (junction 71) : {VVMC_Memory_raw32[VVMC_MemoryShiftCount_enum] =...
        |  VVMC_Memory_raw32[VVMC_RollAveCount_enum - KVMC_WhlSpdRollAveLevel_enum + VVMC_MemoryShiftCount_enum]}
    (junction 25) -> (junction 14)
    (junction 71) -> (junction 73)
    (junction 80) -> (junction 78)
    (junction 45) -> (junction 39) [order 2]
    (junction 45) -> (junction 15) [order 1] : [VVMC_ShiftCount_enum < VVMC_RollAveCount_enum]
    (junction 41) -> (junction 45) : { VVMC_ShiftCount_enum++}
    (junction 15) -> (junction 38) : {% Gy Memory Shift
        |  VVMC_Memory_raw32[VVMC_ShiftCount_enum] = VVMC_Memory_raw32[VVMC_ShiftCount_enum + ONE_INT]}
    (junction 38) -> (junction 41)
  data: KVMC_WhlSpdRollAveLevel_enum input uint8; VVMC_ShiftCount_enum local uint8; VVMC_RollAveCount_enum local uint8; VVMC_Memory_raw32 local single size=100; ZERO_FLOAT input single; ONE_INT input uint8; VVMC_RRWhlSpeedRollAve_kph output single; VINP_RRRawWhlSpeed_kph input single; VVMC_MemoryShiftCount_enum local uint8

== stateflow chart vmc/VMC/VMC/IMU/IMU sensing result /RollingAverage4 ==
  state RollingAverage
    (default) -> (junction 2) : {VVMC_RollAveCount_enum = ONE_INT}
    RollingAverage -> (junction 2)
    (junction 2) -> (junction 3) : {VVMC_RollAve_raw32 = ZERO_FLOAT}
    (junction 3) -> (junction 100) [order 1] : [VVMC_RollAveCount_enum < KVMC_RollAveLevel_enum]
    (junction 3) -> (junction 37) [order 2]
    (junction 100) -> (junction 5) : {% Memory
        |  VVMC_Memory_raw32[VVMC_RollAveCount_enum] = VINP_INPData_raw32;
        |
        |  % Memory Shift Counter
        |  VVMC_ShiftCount_enum = ONE_INT}
    (junction 5) -> (junction 7) [order 2]
    (junction 5) -> (junction 6) [order 1] : [VVMC_ShiftCount_enum <= VVMC_RollAveCount_enum]
    (junction 7) -> (junction 8) : {% Rolling Average
        |  VVMC_RollAve_raw32 = VVMC_RollAve_raw32 / VVMC_RollAveCount_enum;
        |
        |  % Rolling Average Counter
        |  VVMC_RollAveCount_enum++}
    (junction 35) -> (junction 5) : {VVMC_ShiftCount_enum++}
    (junction 6) -> (junction 36) : {% Rolling Average Sum
        |  VVMC_RollAve_raw32 = VVMC_RollAve_raw32 + VVMC_Memory_raw32[VVMC_ShiftCount_enum];
        |  }
    (junction 36) -> (junction 35)
    (junction 37) -> (junction 76) [order 1] : [VVMC_RollAveCount_enum == KVMC_RollAveLevel_enum]
    (junction 76) -> (junction 47)
    (junction 37) -> (junction 60) [order 2]
    (junction 78) -> (junction 76)
    (junction 47) -> (junction 30) : {% Memory
        |  VVMC_Memory_raw32[VVMC_RollAveCount_enum] = VINP_INPData_raw32;
        |
        |  % Memory Shift Counter
        |  VVMC_ShiftCount_enum = ONE_INT;
        | }
    (junction 60) -> (junction 62) [order 1] : [VVMC_RollAveCount_enum > KVMC_RollAveLevel_enum]
    (junction 60) -> (junction 39) [order 2]
    (junction 62) -> (junction 66) : {VVMC_MemoryShiftCount_enum = ONE_INT}
    (junction 30) -> (junction 48) [order 2]
    (junction 30) -> (junction 22) [order 1] : [VVMC_ShiftCount_enum <= VVMC_RollAveCount_enum]
    (junction 48) -> (junction 45) : {% Rolling Average
        |  VVMC_RollAve_raw32 = VVMC_RollAve_raw32 / VVMC_RollAveCount_enum;
        |
        |  % Memory Shift Counter
        |  VVMC_ShiftCount_enum = ONE_INT}
    (junction 14) -> (junction 30) : {VVMC_ShiftCount_enum++}
    (junction 22) -> (junction 25) : {% Rolling Average Sum
        |  VVMC_RollAve_raw32 = VVMC_RollAve_raw32 + VVMC_Memory_raw32[VVMC_ShiftCount_enum]}
    (junction 66) -> (junction 82) [order 2]
    (junction 66) -> (junction 69) [order 1] : [VVMC_MemoryShiftCount_enum < VVMC_RollAveCount_enum]
    (junction 82) -> (junction 80) : {VVMC_RollAveCount_enum = KVMC_RollAveLevel_enum}
    (junction 73) -> (junction 66) : {VVMC_MemoryShiftCount_enum++}
    (junction 69) -> (junction 71) : {VVMC_Memory_raw32[VVMC_MemoryShiftCount_enum] =...
        |  VVMC_Memory_raw32[VVMC_RollAveCount_enum - KVMC_RollAveLevel_enum + VVMC_MemoryShiftCount_enum]}
    (junction 25) -> (junction 14)
    (junction 71) -> (junction 73)
    (junction 80) -> (junction 78)
    (junction 45) -> (junction 39) [order 2]
    (junction 45) -> (junction 15) [order 1] : [VVMC_ShiftCount_enum < VVMC_RollAveCount_enum]
    (junction 41) -> (junction 45) : { VVMC_ShiftCount_enum++}
    (junction 15) -> (junction 38) : {% Gy Memory Shift
        |  VVMC_Memory_raw32[VVMC_ShiftCount_enum] = VVMC_Memory_raw32[VVMC_ShiftCount_enum + ONE_INT]}
    (junction 38) -> (junction 41)
  data: KVMC_RollAveLevel_enum input uint8; VVMC_ShiftCount_enum local uint8; VVMC_RollAveCount_enum local uint8; VVMC_Memory_raw32 local single size=100; ZERO_FLOAT input single; ONE_INT input uint8; VVMC_RollAve_raw32 output single; VINP_INPData_raw32 input single; VVMC_MemoryShiftCount_enum local uint8

== stateflow chart vmc/VMC/VMC/IMU/IMU sensing result /RollingAverage5 ==
  state RollingAverage
    (default) -> (junction 2) : {VVMC_RollAveCount_enum = ONE_INT}
    RollingAverage -> (junction 2)
    (junction 2) -> (junction 3) : {VVMC_RollAve_raw32 = ZERO_FLOAT}
    (junction 3) -> (junction 100) [order 1] : [VVMC_RollAveCount_enum < KVMC_RollAveLevel_enum]
    (junction 3) -> (junction 37) [order 2]
    (junction 100) -> (junction 5) : {% Memory
        |  VVMC_Memory_raw32[VVMC_RollAveCount_enum] = VINP_INPData_raw32;
        |
        |  % Memory Shift Counter
        |  VVMC_ShiftCount_enum = ONE_INT}
    (junction 5) -> (junction 7) [order 2]
    (junction 5) -> (junction 6) [order 1] : [VVMC_ShiftCount_enum <= VVMC_RollAveCount_enum]
    (junction 7) -> (junction 8) : {% Rolling Average
        |  VVMC_RollAve_raw32 = VVMC_RollAve_raw32 / VVMC_RollAveCount_enum;
        |
        |  % Rolling Average Counter
        |  VVMC_RollAveCount_enum++}
    (junction 35) -> (junction 5) : {VVMC_ShiftCount_enum++}
    (junction 6) -> (junction 36) : {% Rolling Average Sum
        |  VVMC_RollAve_raw32 = VVMC_RollAve_raw32 + VVMC_Memory_raw32[VVMC_ShiftCount_enum];
        |  }
    (junction 36) -> (junction 35)
    (junction 37) -> (junction 76) [order 1] : [VVMC_RollAveCount_enum == KVMC_RollAveLevel_enum]
    (junction 76) -> (junction 47)
    (junction 37) -> (junction 60) [order 2]
    (junction 78) -> (junction 76)
    (junction 47) -> (junction 30) : {% Memory
        |  VVMC_Memory_raw32[VVMC_RollAveCount_enum] = VINP_INPData_raw32;
        |
        |  % Memory Shift Counter
        |  VVMC_ShiftCount_enum = ONE_INT;
        | }
    (junction 60) -> (junction 62) [order 1] : [VVMC_RollAveCount_enum > KVMC_RollAveLevel_enum]
    (junction 60) -> (junction 39) [order 2]
    (junction 62) -> (junction 66) : {VVMC_MemoryShiftCount_enum = ONE_INT}
    (junction 30) -> (junction 48) [order 2]
    (junction 30) -> (junction 22) [order 1] : [VVMC_ShiftCount_enum <= VVMC_RollAveCount_enum]
    (junction 48) -> (junction 45) : {% Rolling Average
        |  VVMC_RollAve_raw32 = VVMC_RollAve_raw32 / VVMC_RollAveCount_enum;
        |
        |  % Memory Shift Counter
        |  VVMC_ShiftCount_enum = ONE_INT}
    (junction 14) -> (junction 30) : {VVMC_ShiftCount_enum++}
    (junction 22) -> (junction 25) : {% Rolling Average Sum
        |  VVMC_RollAve_raw32 = VVMC_RollAve_raw32 + VVMC_Memory_raw32[VVMC_ShiftCount_enum]}
    (junction 66) -> (junction 82) [order 2]
    (junction 66) -> (junction 69) [order 1] : [VVMC_MemoryShiftCount_enum < VVMC_RollAveCount_enum]
    (junction 82) -> (junction 80) : {VVMC_RollAveCount_enum = KVMC_RollAveLevel_enum}
    (junction 73) -> (junction 66) : {VVMC_MemoryShiftCount_enum++}
    (junction 69) -> (junction 71) : {VVMC_Memory_raw32[VVMC_MemoryShiftCount_enum] =...
        |  VVMC_Memory_raw32[VVMC_RollAveCount_enum - KVMC_RollAveLevel_enum + VVMC_MemoryShiftCount_enum]}
    (junction 25) -> (junction 14)
    (junction 71) -> (junction 73)
    (junction 80) -> (junction 78)
    (junction 45) -> (junction 39) [order 2]
    (junction 45) -> (junction 15) [order 1] : [VVMC_ShiftCount_enum < VVMC_RollAveCount_enum]
    (junction 41) -> (junction 45) : { VVMC_ShiftCount_enum++}
    (junction 15) -> (junction 38) : {% Gy Memory Shift
        |  VVMC_Memory_raw32[VVMC_ShiftCount_enum] = VVMC_Memory_raw32[VVMC_ShiftCount_enum + ONE_INT]}
    (junction 38) -> (junction 41)
  data: KVMC_RollAveLevel_enum input uint8; VVMC_ShiftCount_enum local uint8; VVMC_RollAveCount_enum local uint8; VVMC_Memory_raw32 local single size=100; ZERO_FLOAT input single; ONE_INT input uint8; VVMC_RollAve_raw32 output single; VINP_INPData_raw32 input single; VVMC_MemoryShiftCount_enum local uint8

== stateflow chart vmc/VMC/VMC/SPD2ACC/ReqACCCalcu/ConstantSpeedControl ==
  state ConstantSpeedControl
    (default) -> (junction 2) : {SpdCtrlFlag = 0;
        |  ReqAccel = 0}
    ConstantSpeedControl -> (junction 2)
    (junction 2) -> (junction 6) [order 1] : [DeltaSpeed >= KVMC_SpdCtrlEnBand_kph && SpdCtrlFlag == 0]
    (junction 2) -> (junction 16) [order 2]
    (junction 6) -> (junction 8) : {SpdCtrlFlag = 1;
        |  ReqAccel = MINUSONE_FLOAT * KVMC_SpdCtrlReqAccel_mps2}
    (junction 16) -> (junction 15) [order 1] : [DeltaSpeed <= MINUSONE_FLOAT * KVMC_SpdCtrlEnBand_kph && SpdCtrlFlag == 0]
    (junction 16) -> (junction 20) [order 2]
    (junction 15) -> (junction 12) : {SpdCtrlFlag = 1;
        |  ReqAccel = KVMC_SpdCtrlReqAccel_mps2}
    (junction 20) -> (junction 18) [order 1] : [SpdCtrlFlag == 1]
    (junction 18) -> (junction 24) [order 1] : [ReqAccel > ZERO_FLOAT]
    (junction 24) -> (junction 26) [order 1] : [DeltaSpeed >= KVMC_SpdCtrlDisBand_kph]
    (junction 20) -> (junction 42) [order 2] : {SpdCtrlFlag = 0}
    (junction 18) -> (junction 40) [order 2]
    (junction 24) -> (junction 30) [order 2] : {SpdCtrlFlag = 1;
        |  ReqAccel = KVMC_SpdCtrlReqAccel_mps2}
    (junction 26) -> (junction 28) : {SpdCtrlFlag = 0;
        |  ReqAccel = ZERO_FLOAT}
    (junction 40) -> (junction 37) [order 1] : [ReqAccel < ZERO_FLOAT]
    (junction 37) -> (junction 33) [order 1] : [DeltaSpeed <= MINUSONE_FLOAT * KVMC_SpdCtrlDisBand_kph]
    (junction 40) -> (junction 49) [order 2]
    (junction 37) -> (junction 35) [order 2] : {SpdCtrlFlag = 1;
        |  ReqAccel = MINUSONE_FLOAT * KVMC_SpdCtrlReqAccel_mps2}
    (junction 33) -> (junction 38) : {SpdCtrlFlag = 0;
        |  ReqAccel = ZERO_FLOAT}
  data: DeltaSpeed input single; SpdCtrlFlag local boolean; ReqAccel output single; KVMC_SpdCtrlEnBand_kph input single; KVMC_SpdCtrlDisBand_kph input single; MINUSONE_FLOAT input single; KVMC_SpdCtrlReqAccel_mps2 input single; ZERO_FLOAT input single

== stateflow chart vmc/VMC/VMC/SafetyControl/SafetyControlJudgement/FrontRearSlipRatio/FrontRearSlipRatioJudgement ==
  state FrontRearSlipRatioJudgement
    (default) -> (junction 14) : {VVMC_FrontRearSlipRatioCtrl_flg = FALSE;
        |  VVMC_FrontAxleWhlSpeedAve_kph = ZERO_FLOAT;
        |  VVMC_RearAxleWhlSpeedAve_kph = ZERO_FLOAT}
    FrontRearSlipRatioJudgement -> (junction 14)
    (junction 14) -> (junction 41) [order 1] : [VINP_LFRawWhlSpeedV_flg == TRUE ||...
        |  VINP_RFRawWhlSpeedV_flg == TRUE]
    (junction 41) -> (junction 69) [order 1] : [VINP_LFRawWhlSpeedV_flg == TRUE &&...
        |  VINP_RFRawWhlSpeedV_flg == TRUE]
    (junction 14) -> (junction 54) [order 2] : {VVMC_FrontAxleWhlSpeedAve_kph =...
        | (VVMC_LFWhlSpeedRollAve_kph+VVMC_RFWhlSpeedRollAve_kph)/TWO_FLOAT}
    (junction 41) -> (junction 52) [order 2]
    (junction 69) -> (junction 47) : {VVMC_FrontRearSlipRatioCtrl_flg = FALSE}
    (junction 52) -> (junction 42) [order 1] : [VINP_LFRawWhlSpeedV_flg == TRUE]
    (junction 52) -> (junction 46) [order 2] : {VVMC_FrontAxleWhlSpeedAve_kph = VVMC_LFWhlSpeedRollAve_kph}
    (junction 42) -> (junction 49) : {VVMC_FrontAxleWhlSpeedAve_kph = VVMC_RFWhlSpeedRollAve_kph}
    (junction 46) -> (junction 54)
    (junction 49) -> (junction 46)
    (junction 54) -> (junction 92)
    (junction 92) -> (junction 85) [order 1] : [VINP_LRRawWhlSpeedV_flg == TRUE ||...
        |  VINP_RRRawWhlSpeedV_flg == TRUE]
    (junction 85) -> (junction 77) [order 1] : [VINP_LRRawWhlSpeedV_flg == TRUE &&...
        |  VINP_RRRawWhlSpeedV_flg == TRUE]
    (junction 92) -> (junction 80) [order 2] : {VVMC_RearAxleWhlSpeedAve_kph =...
        | (VVMC_LRWhlSpeedRollAve_kph+VVMC_RRWhlSpeedRollAve_kph)/TWO_FLOAT}
    (junction 85) -> (junction 89) [order 2]
    (junction 77) -> (junction 79) : {VVMC_FrontRearSlipRatioCtrl_flg = FALSE}
    (junction 89) -> (junction 84) [order 1] : [VINP_LRRawWhlSpeedV_flg == TRUE]
    (junction 89) -> (junction 82) [order 2] : {VVMC_RearAxleWhlSpeedAve_kph = VVMC_LRWhlSpeedRollAve_kph}
    (junction 84) -> (junction 78) : {VVMC_RearAxleWhlSpeedAve_kph = VVMC_RRWhlSpeedRollAve_kph}
    (junction 82) -> (junction 80)
    (junction 78) -> (junction 82)
    (junction 80) -> (junction 96)
    (junction 96) -> (junction 98) [order 1] : [abs(VVMC_RearAxleWhlSpeedAve_kph - VVMC_FrontAxleWhlSpeedAve_kph) >= KVMC_FrontRearSlipRatioTHR_kph]
    (junction 96) -> (junction 103) [order 2] : {VVMC_FrontRearSlipRatioCtrl_flg = FALSE}
    (junction 98) -> (junction 100) : {VVMC_FrontRearSlipRatioCtrl_flg = TRUE}
  data: VVMC_LFWhlSpeedRollAve_kph input single; VVMC_RFWhlSpeedRollAve_kph input single; VVMC_LRWhlSpeedRollAve_kph input single; VVMC_RRWhlSpeedRollAve_kph input single; VINP_LFRawWhlSpeedV_flg input boolean; VINP_RFRawWhlSpeedV_flg input boolean; VINP_LRRawWhlSpeedV_flg input boolean; VINP_RRRawWhlSpeedV_flg input boolean; KVMC_FrontRearSlipRatioTHR_kph input single; TRUE input boolean; VVMC_FrontRearSlipRatioCtrl_flg output boolean; FALSE input boolean; TWO_FLOAT input single; VVMC_FrontAxleWhlSpeedAve_kph local single; ZERO_FLOAT input single; VVMC_RearAxleWhlSpeedAve_kph local single

== stateflow chart vmc/VMC/VMC/IMU/IMU sensing result /RollingAverage ==
  state RollingAverage
    (default) -> (junction 2) : {VVMC_RollAveCount_enum = ONE_INT}
    RollingAverage -> (junction 2)
    (junction 2) -> (junction 3) : {VVMC_RollAve_raw32 = ZERO_FLOAT}
    (junction 3) -> (junction 100) [order 1] : [VVMC_RollAveCount_enum < KVMC_RollAveLevel_enum]
    (junction 3) -> (junction 37) [order 2]
    (junction 100) -> (junction 5) : {% Memory
        |  VVMC_Memory_raw32[VVMC_RollAveCount_enum] = VINP_INPData_raw32;
        |
        |  % Memory Shift Counter
        |  VVMC_ShiftCount_enum = ONE_INT}
    (junction 5) -> (junction 7) [order 2]
    (junction 5) -> (junction 6) [order 1] : [VVMC_ShiftCount_enum <= VVMC_RollAveCount_enum]
    (junction 7) -> (junction 8) : {% Rolling Average
        |  VVMC_RollAve_raw32 = VVMC_RollAve_raw32 / VVMC_RollAveCount_enum;
        |
        |  % Rolling Average Counter
        |  VVMC_RollAveCount_enum++}
    (junction 35) -> (junction 5) : {VVMC_ShiftCount_enum++}
    (junction 6) -> (junction 36) : {% Rolling Average Sum
        |  VVMC_RollAve_raw32 = VVMC_RollAve_raw32 + VVMC_Memory_raw32[VVMC_ShiftCount_enum];
        |  }
    (junction 36) -> (junction 35)
    (junction 37) -> (junction 76) [order 1] : [VVMC_RollAveCount_enum == KVMC_RollAveLevel_enum]
    (junction 76) -> (junction 47)
    (junction 37) -> (junction 60) [order 2]
    (junction 78) -> (junction 76)
    (junction 47) -> (junction 30) : {% Memory
        |  VVMC_Memory_raw32[VVMC_RollAveCount_enum] = VINP_INPData_raw32;
        |
        |  % Memory Shift Counter
        |  VVMC_ShiftCount_enum = ONE_INT;
        | }
    (junction 60) -> (junction 62) [order 1] : [VVMC_RollAveCount_enum > KVMC_RollAveLevel_enum]
    (junction 60) -> (junction 39) [order 2]
    (junction 62) -> (junction 66) : {VVMC_MemoryShiftCount_enum = ONE_INT}
    (junction 30) -> (junction 48) [order 2]
    (junction 30) -> (junction 22) [order 1] : [VVMC_ShiftCount_enum <= VVMC_RollAveCount_enum]
    (junction 48) -> (junction 45) : {% Rolling Average
        |  VVMC_RollAve_raw32 = VVMC_RollAve_raw32 / VVMC_RollAveCount_enum;
        |
        |  % Memory Shift Counter
        |  VVMC_ShiftCount_enum = ONE_INT}
    (junction 14) -> (junction 30) : {VVMC_ShiftCount_enum++}
    (junction 22) -> (junction 25) : {% Rolling Average Sum
        |  VVMC_RollAve_raw32 = VVMC_RollAve_raw32 + VVMC_Memory_raw32[VVMC_ShiftCount_enum]}
    (junction 66) -> (junction 82) [order 2]
    (junction 66) -> (junction 69) [order 1] : [VVMC_MemoryShiftCount_enum < VVMC_RollAveCount_enum]
    (junction 82) -> (junction 80) : {VVMC_RollAveCount_enum = KVMC_RollAveLevel_enum}
    (junction 73) -> (junction 66) : {VVMC_MemoryShiftCount_enum++}
    (junction 69) -> (junction 71) : {VVMC_Memory_raw32[VVMC_MemoryShiftCount_enum] =...
        |  VVMC_Memory_raw32[VVMC_RollAveCount_enum - KVMC_RollAveLevel_enum + VVMC_MemoryShiftCount_enum]}
    (junction 25) -> (junction 14)
    (junction 71) -> (junction 73)
    (junction 80) -> (junction 78)
    (junction 45) -> (junction 39) [order 2]
    (junction 45) -> (junction 15) [order 1] : [VVMC_ShiftCount_enum < VVMC_RollAveCount_enum]
    (junction 41) -> (junction 45) : { VVMC_ShiftCount_enum++}
    (junction 15) -> (junction 38) : {% Gy Memory Shift
        |  VVMC_Memory_raw32[VVMC_ShiftCount_enum] = VVMC_Memory_raw32[VVMC_ShiftCount_enum + ONE_INT]}
    (junction 38) -> (junction 41)
  data: KVMC_RollAveLevel_enum input uint8; VVMC_ShiftCount_enum local uint8; VVMC_RollAveCount_enum local uint8; VVMC_Memory_raw32 local single size=100; ZERO_FLOAT input single; ONE_INT input uint8; VVMC_RollAve_raw32 output single; VINP_INPData_raw32 input single; VVMC_MemoryShiftCount_enum local uint8

== stateflow chart vmc/VMC/VMC/SafetyControl/SafetyControlJudgement/RearWheelSlipRatio/FrontRearSlipRatioJudgement ==
  state RearWheelSlipRatioJudgement
    (default) -> (junction 14) : {VVMC_RearWhlSlipRatioCtrl_flg = FALSE}
    RearWheelSlipRatioJudgement -> (junction 14)
    (junction 14) -> (junction 85) [order 1] : [VINP_LRRawWhlSpeedV_flg == TRUE ||...
        |  VINP_RRRawWhlSpeedV_flg == TRUE]
    (junction 14) -> (junction 96) [order 2]
    (junction 85) -> (junction 105) : {VVMC_RearWhlSlipRatioCtrl_flg = FALSE}
    (junction 96) -> (junction 98) [order 1] : [abs(VVMC_LRWhlSpeedRollAve_kph - VVMC_RRWhlSpeedRollAve_kph) >= KVMC_RearWhlSlipRatioTHR_kph]
    (junction 96) -> (junction 103) [order 2] : {VVMC_RearWhlSlipRatioCtrl_flg = FALSE}
    (junction 98) -> (junction 100) : {VVMC_RearWhlSlipRatioCtrl_flg = TRUE}
  data: VVMC_LRWhlSpeedRollAve_kph input single; VVMC_RRWhlSpeedRollAve_kph input single; VINP_LRRawWhlSpeedV_flg input boolean; VINP_RRRawWhlSpeedV_flg input boolean; KVMC_RearWhlSlipRatioTHR_kph input single; TRUE input boolean; VVMC_RearWhlSlipRatioCtrl_flg output boolean; FALSE input boolean
